simulink model "model_1"  (R2022a)
settings: Solver=VariableStepAuto  StartTime=0.0  StopTime=12  RelTol=1e-3
values from neighbouring files (symbols this model uses):
  A = [6, 7, -4, 8; 0, 9, 0, 15; 10, 13, -6, 19; 0, -6, 0, -9]    [task_2.m]
  B = [-8, 0; 4, 0; -6, 0; -2, 0]    [task_2.m]
  C = eye(4)    [task_2.m]
  D = zeros(4, 2)    [task_2.m]
  K_1 = -K_1    [task_2.m]
  K_2 = Y*inv(P)    [task_2.m]
  K_3 = Y*inv(P)    [task_2.m]
  x0 = [1; -1; 1; -1]    [task_2.m]
settings Model: Creator=vital  LastModifiedBy=Family
settings DebuggingCC: UnconnectedInputMsg=warning  UnconnectedOutputMsg=warning  UnconnectedLineMsg=warning
settings RTWCC: DLArmComputeVersion=19.05

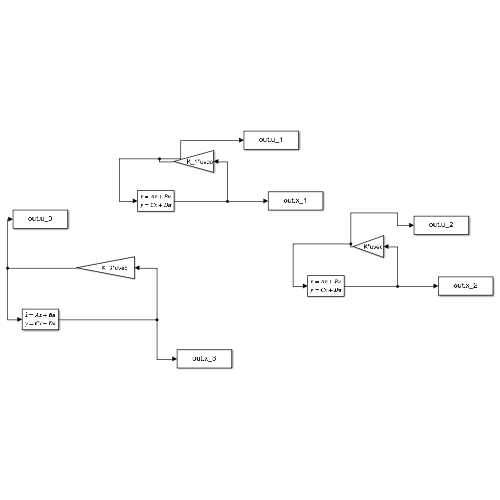
[thumbnail: Simulink's stored preview of the top-level diagram]
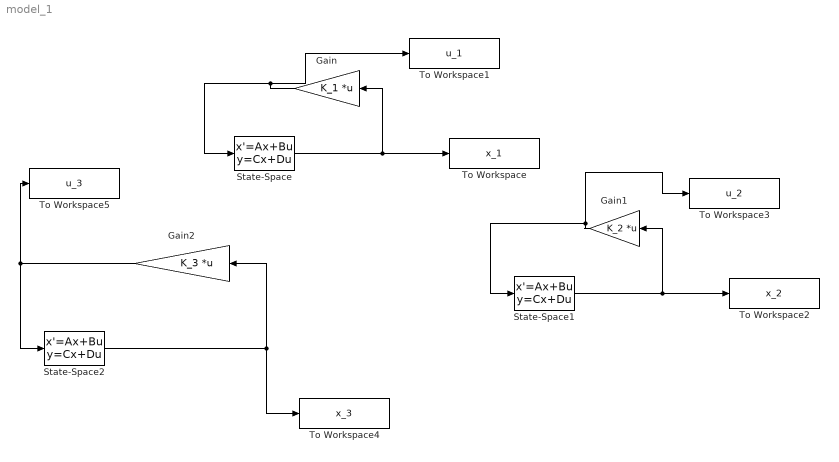
== system model_1 ==
  Gain : Gain  Gain=K_1  Multiplication=Matrix(K*u) (u vector)
  Gain1 : Gain  Gain=K_2  Multiplication=Matrix(K*u) (u vector)
  Gain2 : Gain  Gain=K_3  Multiplication=Matrix(K*u) (u vector)
  State-Space : StateSpace  A=A  B=B  C=C  D=D  InitialCondition=x0  ParameterTunability=Optimized
  State-Space1 : StateSpace  A=A  B=B  C=C  D=D  InitialCondition=x0  ParameterTunability=Unconstrained
  State-Space2 : StateSpace  A=A  B=B  C=C  D=D  InitialCondition=x0  ParameterTunability=Optimized
  To Workspace : ToWorkspace  VariableName=x_1  SaveFormat=Timeseries  SampleTime=-1
  To Workspace1 : ToWorkspace  VariableName=u_1  SaveFormat=Timeseries  SampleTime=0.00001
  To Workspace2 : ToWorkspace  VariableName=x_2  SaveFormat=Timeseries  SampleTime=-1
  To Workspace3 : ToWorkspace  VariableName=u_2  SaveFormat=Timeseries  SampleTime=0.00001
  To Workspace4 : ToWorkspace  VariableName=x_3  SaveFormat=Timeseries  SampleTime=-1
  To Workspace5 : ToWorkspace  VariableName=u_3  SaveFormat=Timeseries  SampleTime=0.00001
  wires:
  State-Space/1 -> Gain/1, To Workspace/1
  State-Space2/1 -> Gain2/1, To Workspace4/1
  Gain1/1 -> To Workspace3/1, State-Space1/1
  State-Space1/1 -> Gain1/1, To Workspace2/1
  Gain/1 -> To Workspace1/1, State-Space/1
  Gain2/1 -> To Workspace5/1, State-Space2/1
